simulink model "test_identification"  (Simulink 6.5)
settings: Solver=ode45  StartTime=0.0  StopTime=L  RelTol=1e-6
undefined symbols (not defined in the file or in its folder): Delta, fr, Ig, K, Ktach, L, M_ecart, N, Tc, Te
settings Model: Creator=admin  LastModifiedBy=admin
settings DataIOCC: SignalLoggingName=sigsOut
settings DebuggingCC: SolverPrmCheckMsg=none  MultiTaskDSMMsg=warning  MultiTaskCondExecSysMsg=none  StrictBusMsg=None
settings HardwareCC: TargetUnknown=on
settings RTWCC: IncludeERTFirstTime=on

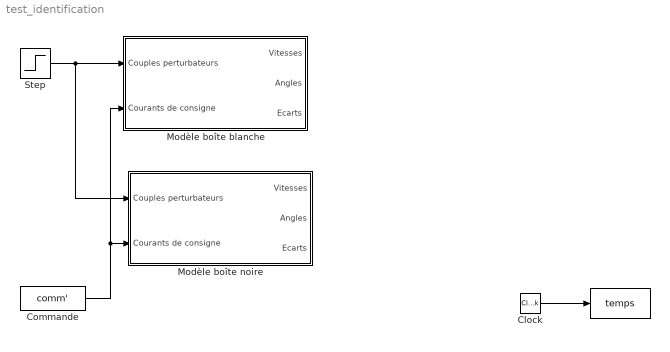
== system test_identification ==
  " " : ToWorkspace  VariableName=temps  SampleTime=-1  SaveFormat=Array
  Clock : DigitalClock  SampleTime=Te
  Commande : FromWorkspace  VariableName=comm'  SampleTime=Tc
  Modèle boîte blanche : Subsystem
  Modèle boîte noire : Subsystem
  Step : Step  Time=L*0.1  Before=zeros(N,1)  After=zeros(N,1)
  wires:
  Step/1 -> Modèle boîte blanche/1(Couples perturbateurs), Modèle boîte noire/1(Couples perturbateurs)
  Clock/1 -> " "/1
  Commande/1 -> Modèle boîte blanche/2(Courants de consigne), Modèle boîte noire/2(Courants de consigne)

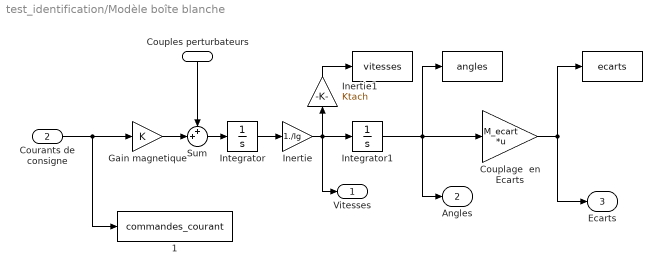
== system test_identification/Modèle boîte blanche ==
  Couples perturbateurs : Inport  Orientation=down
  Courants de consigne : Inport  Port=2
  " " : ToWorkspace  VariableName=vitesses  SampleTime=Te  SaveFormat=Array
  "  " : ToWorkspace  VariableName=angles  SampleTime=Te  SaveFormat=Array
  "   " : ToWorkspace  VariableName=ecarts  SampleTime=Te  SaveFormat=Array
  "   1" : ToWorkspace  VariableName=commandes_courant  SampleTime=-1  SaveFormat=Array
  Couplage  en Ecarts : Gain  Gain=M_ecart  Multiplication=Matrix(K*u)  SaturateOnIntegerOverflow=on
  Gain magnetique : Gain  Gain=K  SaturateOnIntegerOverflow=on
  Inertie : Gain  Gain=1./Ig  SaturateOnIntegerOverflow=on
  Inertie1 : Gain  Orientation=up  Gain=Ktach  SaturateOnIntegerOverflow=on
  Integrator : Integrator  InitialCondition=zeros(N,1)
  Integrator1 : Integrator  InitialCondition=(0:N-1)*Delta
  Sum : Sum  Inputs=++|  SaturateOnIntegerOverflow=on
  Vitesses : Outport
  Angles : Outport  Port=2
  Ecarts : Outport  Port=3
  wires:
  Integrator/1 -> Inertie/1
  Gain magnetique/1 -> Sum/2
  Sum/1 -> Integrator/1
  Integrator1/1 -> "  "/1, Angles/1, Couplage  en Ecarts/1
  Couples perturbateurs/1 -> Sum/1
  Courants de consigne/1 -> Gain magnetique/1, "   1"/1
  Couplage  en Ecarts/1 -> "   "/1, Ecarts/1
  Inertie/1 -> Vitesses/1, Inertie1/1, Integrator1/1
  Inertie1/1 -> " "/1

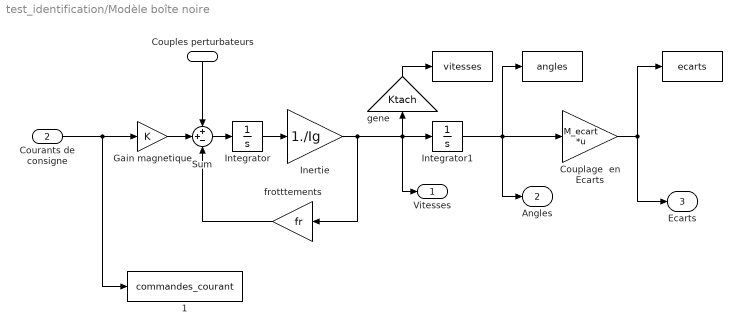
== system test_identification/Modèle boîte noire ==
  Couples perturbateurs : Inport  Orientation=down
  Courants de consigne : Inport  Port=2
  " " : ToWorkspace  VariableName=vitesses  SampleTime=Te  SaveFormat=Array
  "  " : ToWorkspace  VariableName=angles  SampleTime=Te  SaveFormat=Array
  "   " : ToWorkspace  VariableName=ecarts  SampleTime=Te  SaveFormat=Array
  "   1" : ToWorkspace  VariableName=commandes_courant  SampleTime=-1  SaveFormat=Array
  Couplage  en Ecarts : Gain  Gain=M_ecart  Multiplication=Matrix(K*u)  SaturateOnIntegerOverflow=on
  Gain magnetique : Gain  Gain=K  SaturateOnIntegerOverflow=on
  Inertie : Gain  Gain=1./Ig  SaturateOnIntegerOverflow=on
  Integrator : Integrator  InitialCondition=zeros(N,1)
  Integrator1 : Integrator  InitialCondition=(0:N-1)*Delta
  Sum : Sum  Inputs=++-  SaturateOnIntegerOverflow=on
  frotttements : Gain  Orientation=left  Gain=fr  SaturateOnIntegerOverflow=on
  gene : Gain  Orientation=up  Gain=Ktach  SaturateOnIntegerOverflow=on
  Vitesses : Outport
  Angles : Outport  Port=2
  Ecarts : Outport  Port=3
  wires:
  gene/1 -> " "/1
  Inertie/1 -> Integrator1/1, gene/1, Vitesses/1, frotttements/1
  Couplage  en Ecarts/1 -> Ecarts/1, "   "/1
  Courants de consigne/1 -> "   1"/1, Gain magnetique/1
  Couples perturbateurs/1 -> Sum/1
  Integrator1/1 -> Couplage  en Ecarts/1, Angles/1, "  "/1
  Sum/1 -> Integrator/1
  Gain magnetique/1 -> Sum/2
  Integrator/1 -> Inertie/1
  frotttements/1 -> Sum/3
